simulink subsystem "StudentTemplate_M2_DRAFT3"  (R2025a)
settings: Solver=VariableStepAuto  StartTime=0.0  StopTime=10.0  RelTol=1e-3
libraries: simulink x5, eeGeneralControl x3, slpidlib x3
settings Model: Creator=JesseJabezArendse  LastModifiedBy=MTMTAD006

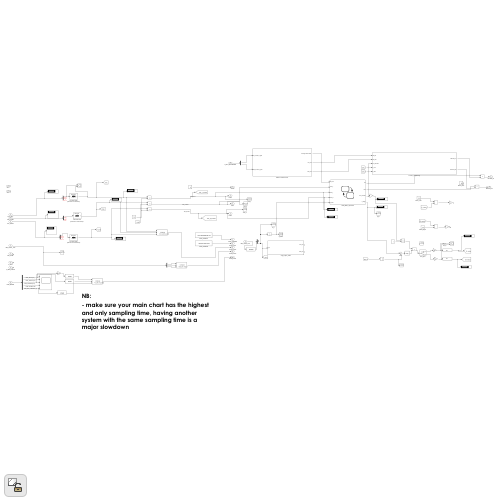
[thumbnail: Simulink's stored preview of the top-level diagram]
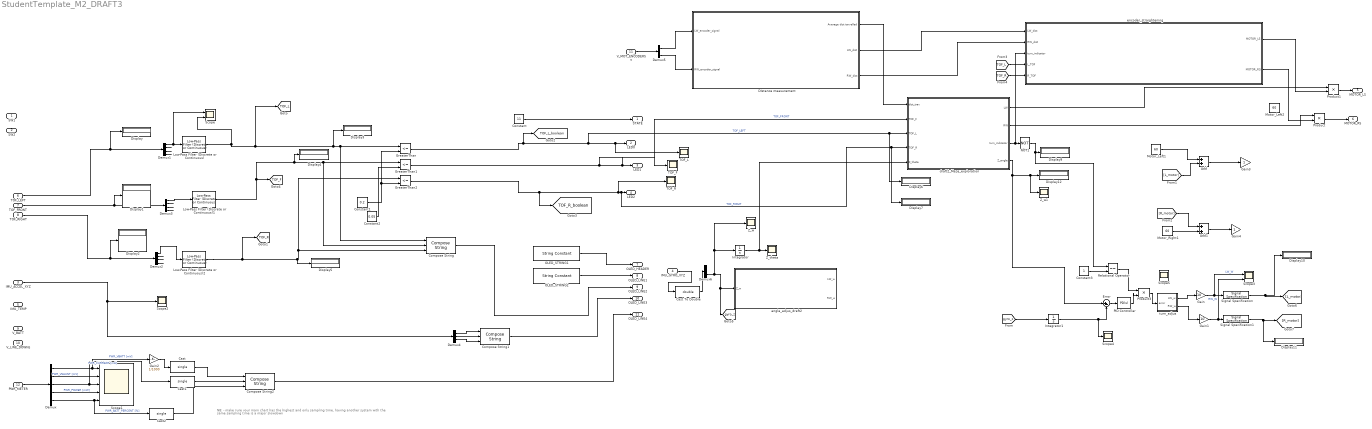
== system StudentTemplate_M2_DRAFT3 ==
  note: NB:
      |
      | - make sure your main chart has the highest and only sampling time, having another system with the same sampling time is a major slowdown
  SW1 : Inport
  SW2 : Inport  Port=2
  IMU_ACCEL_XYZ : Inport  Port=3
  IMU_GYRO_XYZ : Inport  Port=4
  IMU_TEMP : Inport  Port=5
  TOF_LEFT : Inport  Port=6
  TOF_FRONT : Inport  Port=7
  TOF_RIGHT : Inport  Port=8
  V_BATT : Inport  Port=9
  V_LINE_DOWNs : Inport  Port=10
  V_MOT_ENCODERSs : Inport  Port=11
  PWR_METER : Inport  Port=12
  Add : Sum
  Add1 : Sum
  Cast : DataTypeConversion  OutDataTypeStr=single  SaturateOnIntegerOverflow=off  RndMeth=Floor
  Cast To Double : DataTypeConversion  OutDataTypeStr=double  SaturateOnIntegerOverflow=off  RndMeth=Floor
  Cast1 : DataTypeConversion  OutDataTypeStr=single  SaturateOnIntegerOverflow=off  RndMeth=Floor
  Cast2 : DataTypeConversion  OutDataTypeStr=single  SaturateOnIntegerOverflow=off  RndMeth=Floor
  Compose String : ComposeString  Format="\"L%1.2f F%1.2f R%1.2f\""
  Compose String1 : ComposeString  Format="\"X%2.1f  Y%2.1f  Z%2.1f\""
  Compose String2 : ComposeString  Format="\"%1.2fV  %3.0fmA  %2.0f%%\""
  Constant : Constant  Value=11
  Constant1 : Constant  Value=0.2  SampleTime=-1
  Constant2 : Constant  Value=0.05  SampleTime=-1
  Constant3 : Constant
  "DIstance measurement " : Subsystem
  Demux : Demux  Outputs=5
  Demux1 : Demux
  Demux2 : Demux
  Demux3 : Demux
  Demux4 : Demux  Outputs=3
  Demux5 : Demux  Outputs=2
  Demux6 : Demux  Outputs=3
  Display{,1..7,9..12} (12 alike) : Display
  Error : Sum  Inputs=|+-
  Gain : Gain  Gain=10
  Gain1 : Gain  Gain=10
  Gain2 : Gain  Gain=1/1000
  Gain3 : Gain
  Gain4 : Gain
  GreaterThan : RelationalOperator  Operator=<=  OutDataTypeStr=boolean  RndMeth=Simplest  InputSameDT=off
  GreaterThan1 : RelationalOperator  Operator=<=  OutDataTypeStr=boolean  RndMeth=Simplest  InputSameDT=off
  GreaterThan2 : RelationalOperator  Operator=<=  OutDataTypeStr=boolean  RndMeth=Simplest  InputSameDT=off
  Integrator : Integrator
  Integrator1 : Integrator
  Low-Pass Filter (Discrete or Continuous) : eeGeneralControl/Low-Pass Filter (Discrete or Continuous)  K=1  T=0.1  B=inf  A=-inf  init_option=Inherited from block input  x0=0  Ts=-1
  Low-Pass Filter (Discrete or Continuous)1 : eeGeneralControl/Low-Pass Filter (Discrete or Continuous)  K=1  T=0.1  B=inf  A=-inf  init_option=Inherited from block input  x0=0  Ts=-1
  Low-Pass Filter (Discrete or Continuous)2 : eeGeneralControl/Low-Pass Filter (Discrete or Continuous)  K=1  T=0.1  B=inf  A=-inf  init_option=Inherited from block input  x0=0  Ts=-1
  Motor_Left1 : Constant  Value=60
  Motor_Left2 : Constant  Value=60
  Motor_Right1 : Constant  Value=60
  NOT1 : Logic  Operator=NOT  IconShape=distinctive  AllPortsSameDT=off  OutDataTypeStr=boolean
  OLED_STRING1 : StringConstant  String="\"UCT MICROMOUSE '25\""
  OLED_STRING2 : StringConstant  String="\"Simulink Data Demo\""
  PID Controller : slpidlib/PID Controller  Controller=PD  Form=Parallel  TimeDomain=Continuous-time  UseExternalTs=off  SampleTime=-1  IntegratorMethod=Forward Euler  FilterMethod=Forward Euler  ControllerParametersSource=internal  P=50  I=1  UseKiTs=off  D=1  UseExternalDerivativeSource=off  N=100  UseFilter=on  TunerSelectOption=Transfer Function Based (PID Tuner App)  InitialConditionSource=internal  InitialConditionForIntegrator=0  InitialConditionForFilter=0  DifferentiatorICPrevScaledInput=0  ExternalReset=none  TrackingMode=off  Kt=1  LimitOutput=off  SatLimitsSource=internal  UpperSaturationLimit=inf  LowerSaturationLimit=-inf  LinearizeAsGain=on  AntiWindupMode=none  Kb=1  LimitIntegrator=off  UpperIntegratorSaturationLimit=inf  LowerIntegratorSaturationLimit=-inf  POutMin=[]  POutMax=[]  IOutMin=[]  IOutMax=[]  DOutMin=[]  DOutMax=[]  NOutMin=[]  NOutMax=[]  SumOutMin=[]  SumOutMax=[]  SaturationOutMin=[]  SaturationOutMax=[]  PParamMin=[]  PParamMax=[]  IParamMin=[]  IParamMax=[]  DParamMin=[]  DParamMax=[]  NParamMin=[]  NParamMax=[]  KbParamMin=[]  KbParamMax=[]  KtParamMin=[]  KtParamMax=[]  KbOutMin=[]  KbOutMax=[]  KtOutMin=[]  KtOutMax=[]  IntegratorOutMin=[]  IntegratorOutMax=[]  FilterOutMin=[]  FilterOutMax=[]  SumI1OutMin=[]  SumI1OutMax=[]  SumI2OutMin=[]  SumI2OutMax=[]  SumI3OutMin=[]  SumI3OutMax=[]  SumI4OutMin=[]  SumI4OutMax=[]  SumDOutMin=[]  SumDOutMax=[]  DifferentiatorOutMin=[]  DifferentiatorOutMax=[]  FilterDiffOutCoefMin=[]  FilterDiffOutCoefMax=[]  ReciprocalOutMin=[]  ReciprocalOutMax=[]  SumDenOutMin=[]  SumDenOutMax=[]  SumNumOutMin=[]  SumNumOutMax=[]  DivideOutMin=[]  DivideOutMax=[]  UdiffTsProdOutMin=[]  UdiffTsProdOutMax=[]  NTsProdOutMin=[]  NTsProdOutMax=[]  UintegralTsProdOutMin=[]  UintegralTsProdOutMax=[]  UngainTsProdOutMin=[]  UngainTsProdOutMax=[]  ClampingZeroOutDataTypeStr=Inherit: Inherit via back propagation  ClampingZeroOutMin=[]  ClampingZeroOutMax=[]  FilterDenConstantOutDataTypeStr=Inherit: Inherit via back propagation  FilterDenConstantOutMin=[]  FilterDenConstantOutMax=[]  PCopyOutDataTypeStr=Inherit: Inherit via back propagation  PCopyOutMin=[]  PCopyOutMax=[]  NCopyOutDataTypeStr=Inherit: Inherit via back propagation  NCopyOutMin=[]  NCopyOutMax=[]  IntegratorContinuousStateAttributes=''  IntegratorStateMustResolveToSignalObject=off  IntegratorRTWStateStorageClass=Auto  FilterContinuousStateAttributes=''  FilterStateMustResolveToSignalObject=off  FilterRTWStateStorageClass=Auto  ParallelPVariant=InternalParameters  IdealPVariant=Disabled  IVariant=Disabled  DVariant=InternalParameters  IntegratorVariant=Disabled  SatVariant=Disabled  AWVariant=Disabled  PCopyVariant=Disabled  TRVariant=Disabled  FdbkBlocksVariant=Forward  IdealPFdbkVariant=Disabled  SatFdbkVariant=Disabled  DerivativeFilterVariant=ContFilter  NVariant=InternalParameters  NCopyVariant=Disabled  FilterICVariant=InternalICsFilter  IntegratorICVariant=Disabled  ExternalResetVariant=Disabled  TRSumVariant=Passthrough  SumFdbkVariant=Disabled  SumVariant=Sum_PD  TsampFilterVariant=InternalTs  TsampNgainVariant=Passthrough  TsampIntegralVariant=Disabled_SignalSpec  ExternalSaturationOutDataTypeStr=Inherit: Same as second input  DerivativeSourceVariant=ErrorSignal  PreIntVariant=InternalPreInt
  Product : Product
  Product1 : Product
  Product3 : Product
  Relational Operator : RelationalOperator  Operator===  OutDataTypeStr=boolean  RndMeth=Simplest  InputSameDT=off
  Scope : Scope  NumInputPorts=2
      settings: ActiveDisplayYMinimum=0.15223708238283273  ActiveDisplayYMaximum=0.58543478513497516
  Scope1 : Scope  NumInputPorts=5
      settings: ActiveDisplayYMinimum=-437.5  ActiveDisplayYMaximum=3937.5  DataLoggingVariableName=ScopeData2
  Scope2 : Scope
      settings: ActiveDisplayYMinimum=-7.57059273149099  ActiveDisplayYMaximum=14.477362665673041
  Scope3 : Scope  NumInputPorts=2
      settings: ActiveDisplayYMinimum=-440.40684872460486  ActiveDisplayYMaximum=398.93122569343797  DataLoggingVariableName=ScopeData11
  Scope4 : Scope
      settings: ActiveDisplayYMinimum=-2.1976138852237335  ActiveDisplayYMaximum=0.12970641062525379  DataLoggingVariableName=ScopeData14
  Scope5 : Scope
      settings: ActiveDisplayYMinimum=-4.4488284675734473  ActiveDisplayYMaximum=3.9249085751009725  DataLoggingVariableName=ScopeData16
  Signal Specification : SignalSpecification  Dimensions=1
  Signal Specification1 : SignalSpecification  Dimensions=1
  TOF_F : Scope
      settings: ActiveDisplayYMinimum=-0.1769980412947128  ActiveDisplayYMaximum=0.90279895686963285  DataLoggingVariableName=ScopeData4
  TOF_L : Scope
      settings: ActiveDisplayYMinimum=-0.062899688908756052  ActiveDisplayYMaximum=0.13734742485444948  DataLoggingVariableName=ScopeData3
  TOF_R : Scope
      settings: ActiveDisplayYMinimum=0.84085955530656642  ActiveDisplayYMaximum=1.1222796398378163  DataLoggingVariableName=ScopeData5
  Z_theta : Scope
      settings: ActiveDisplayYMinimum=-2.70161604115423  ActiveDisplayYMaximum=4.8892356554264911  DataLoggingVariableName=ScopeData7
  Z_w : Scope
      settings: ActiveDisplayYMinimum=0.15654767663707053  ActiveDisplayYMaximum=0.20860795869615065  DataLoggingVariableName=ScopeData6
  Z_w1 : Scope
      settings: ActiveDisplayYMinimum=0.15654767663707053  ActiveDisplayYMaximum=0.20860795869615065  DataLoggingVariableName=ScopeData25
  angle_adjus_draft2 : Subsystem
  draft2_Maze_exploration : Stateflow chart  TreatAsAtomicUnit=on
      settings: PortSchema="{\"entries\":[{\"content\":{\"sides\":[{\"content\":{\"connectorIds\":[\"In3\",\"In4\",\"In1\",\"In2\",\"In5\"]},\"type\":\"ConnectorPlacement.EquallySpacedRectSide\",\"uuid\":\"48a59af2-7c84-427a-8e2f-b10f2a044ed3\"},{\"content\":{\"connectorIds\":[\"Out1\",\"Out2\",\"Out3\",\"Out4\"],\"side\":\"RIGHT\"},\"type\":\"ConnectorPlacement.EquallySpacedRectSide\",\"uuid\":\"ddb5ed95-9874-42e8-8fee-75458ccb7c53\"},{\"content\":{\"side\":\"TOP\"},\"type\":\"ConnectorPlacement.EquallySpacedRectSide\",\"uuid\":\"d57417fe-864c-49b1-b704-1964fc5ecc42\"}]},\"type\":\"ConnectorPlacement.EquallySpacedConnector\",\"uuid\":\"f24c4a6d-faf6-462a-ab68-e289d44b6927\"}],\"packageUris\":[\"http://schema.mathworks.com/mf0/Connector/R2020b\"],\"version\":\"1.0\"}"
  encoder_straightening : Subsystem
  turn_adjus : Stateflow chart  TreatAsAtomicUnit=on
  STATE : Outport
  LED0 : Outport  Port=2
  LED1 : Outport  Port=3
  LED2 : Outport  Port=4
  MOTOR_LS : Outport  Port=5
  MOTOR_RS : Outport  Port=6
  OLED_HEADER : Outport  Port=7
  OLED_LINE1 : Outport  Port=8
  OLED_LINE2 : Outport  Port=9
  OLED_LINE3 : Outport  Port=10
  OLED_LINE4 : Outport  Port=11
  tag scope: TOF_F=global, TOF_L=global, TOF_L_boolean=global, TOF_R=global, TOF_R_boolean=global, gyro_z=global
  wires:
  TOF_FRONT/1 -> Demux3/1, Display1/1
  OLED_STRING2/1 -> OLED_LINE1/1
  Demux2/1 -> Low-Pass Filter (Discrete or Continuous)2/1
  Demux2/3 -> ?
  Demux2/2 -> ?
  Demux2/4 -> ?
  Compose String1/1 -> OLED_LINE3/1
  Low-Pass Filter (Discrete or Continuous)1/1 -> [TOF_F], Compose String/2, GreaterThan1/1, Display4/1
  GreaterThan1/1 -> LED1/1, TOF_F/1, draft2_Maze_exploration/4(TOF_F)  "TOF_FRONT"
  Demux3/3 -> ?
  TOF_RIGHT/1 -> Demux2/1, Display2/1
  Demux3/4 -> ?
  Demux3/2 -> ?
  Demux1/2 -> ?
  Demux3/1 -> Low-Pass Filter (Discrete or Continuous)1/1
  OLED_STRING1/1 -> OLED_HEADER/1
  Demux1/1 -> Scope/1, Low-Pass Filter (Discrete or Continuous)/1
  Compose String/1 -> OLED_LINE2/1
  Constant1/1 -> GreaterThan2/2, GreaterThan/2
  Demux1/4 -> ?
  GreaterThan2/1 -> TOF_R/1, LED2/1, draft2_Maze_exploration/2(TOF_R), Display7/1, [TOF_R_boolean]  "TOF_RIGHT"
  TOF_LEFT/1 -> Demux1/1, Display/1
  GreaterThan/1 -> LED0/1, TOF_L/1, draft2_Maze_exploration/1(TOF_L), Display6/1, [TOF_L_boolean]  "TOF_LEFT"
  Demux1/3 -> ?
  PWR_METER/1 -> Demux/1
  Demux/1 -> Scope1/1, Gain2/1  "PWR_VBATT [mV]"
  Demux/2 -> Scope1/2  "PWR_VSHUNT [mV]"
  Demux/3 -> Scope1/3, Cast1/1  "PWR_CURRENT [mA]"
  Demux/4 -> Scope1/4  "PWR_POWER [mW]"
  Demux/5 -> Scope1/5, Cast2/1  "PWR_BATT_PERCENT [%]"
  IMU_ACCEL_XYZ/1 -> Demux4/1, Scope2/1
  Demux4/1 -> Compose String1/1
  Demux4/2 -> Compose String1/2
  Demux4/3 -> Compose String1/3
  Compose String2/1 -> OLED_LINE4/1
  Gain2/1 -> Cast/1
  Cast/1 -> Compose String2/1
  Cast1/1 -> Compose String2/2
  Cast2/1 -> Compose String2/3
  Low-Pass Filter (Discrete or Continuous)2/1 -> Compose String/3, GreaterThan2/1, Display5/1, [TOF_R]
  Low-Pass Filter (Discrete or Continuous)/1 -> Scope/2, Compose String/1, GreaterThan/1, Display3/1, [TOF_L]
  Constant/1 -> STATE/1
  V_MOT_ENCODERSs/1 -> Demux5/1
  Demux5/1 -> "DIstance measurement "/1(LW_encoder_signal)
  Demux5/2 -> "DIstance measurement "/2(RW_encoder_signal)
  IMU_GYRO_XYZ/1 -> Cast To Double/1
  Demux6/3 -> angle_adjus_draft2/1(Z_w), [gyro_z], Integrator/1, Z_w/1
  Integrator/1 -> Z_theta/1, draft2_Maze_exploration/5(Z_theta)
  Error/1 -> PID Controller/1
  Signal Specification/1 -> [L_motor], Display10/1
  turn_adjus/1(LW_w) -> Gain/1
  turn_adjus/2(RW_w) -> Gain1/1
  Gain1/1 -> Signal Specification1/1, Scope3/2  "RW_W"
  Integrator1/1 -> Error/2, Scope4/1
  Signal Specification1/1 -> [R_motor], Display11/1
  Gain/1 -> Signal Specification/1, Scope3/1  "LW_W"
  Constant2/1 -> GreaterThan1/2
  draft2_Maze_exploration/1(LW) -> Product1/1
  draft2_Maze_exploration/2(RW) -> Product/1
  Motor_Left1/1 -> Add/1
  Motor_Right1/1 -> Add1/2
  Add/1 -> Gain3/1
  Add1/1 -> Gain4/1
  "DIstance measurement "/1("Average dist tarvelled ") -> draft2_Maze_exploration/3(dist_trav)
  [gyro_z] -> Integrator1/1
  draft2_Maze_exploration/4(Z_angle) -> Error/1, Z_w1/1, Display12/1
  [L_motor] -> Add/2
  [R_motor] -> Add1/1
  draft2_Maze_exploration/3(turn_indicator) -> NOT1/1, encoder_straightening/3(turn_indicator)
  NOT1/1 -> Display9/1, Relational Operator/1
  Constant3/1 -> Relational Operator/2
  PID Controller/1 -> Product3/2
  Product3/1 -> turn_adjus/1(error)
  Relational Operator/1 -> Product3/1
  "DIstance measurement "/2(LW_dist) -> encoder_straightening/1(LW_dist)
  "DIstance measurement "/3(RW_dist) -> encoder_straightening/2(RW_dist)
  [TOF_L] -> encoder_straightening/4(L_TOF)
  [TOF_R] -> encoder_straightening/5(R_TOF)
  Cast To Double/1 -> Demux6/1
  Product1/1 -> MOTOR_LS/1
  Product/1 -> MOTOR_RS/1
  encoder_straightening/1(MOTOR_LS) -> Product1/2
  encoder_straightening/2(MOTOR_RS) -> Product/2

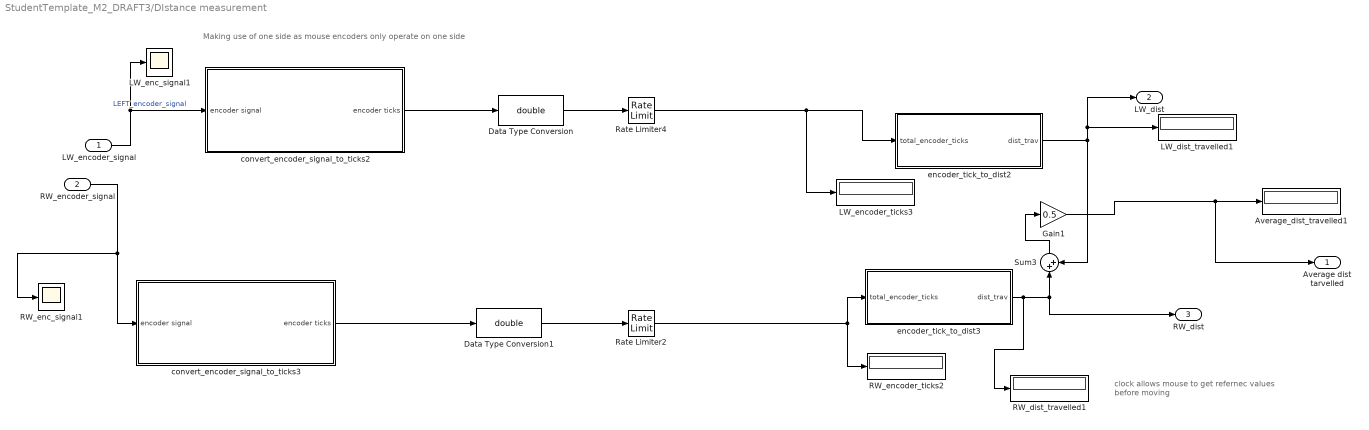
== system StudentTemplate_M2_DRAFT3/DIstance measurement  ==
  note: Making use of one side as mouse encoders only operate on one side
  note: clock allows mouse to get refernec values
      | before moving
  LW_encoder_signal : Inport
  RW_encoder_signal : Inport  Port=2
  Average_dist_travelled1 : Display
  Data Type Conversion : DataTypeConversion  OutDataTypeStr=double  SaturateOnIntegerOverflow=off  RndMeth=Floor
  Data Type Conversion1 : DataTypeConversion  OutDataTypeStr=double  SaturateOnIntegerOverflow=off  RndMeth=Floor
  Gain1 : Gain  Gain=0.5
  LW_dist_travelled1 : Display
  LW_enc_signal1 : Scope
      settings: ActiveDisplayYMinimum=-1.5423087408726712  ActiveDisplayYMaximum=1.7466656009006407  DataLoggingVariableName=ScopeData13
  LW_encoder_ticks3 : Display
  RW_dist_travelled1 : Display
  RW_enc_signal1 : Scope
      settings: ActiveDisplayYMinimum=-1.944570956862778  ActiveDisplayYMaximum=2.0482644886882531  DataLoggingVariableName=ScopeData15
  RW_encoder_ticks2 : Display
  Rate Limiter2 : RateLimiter  RisingSlewLimit=4.85
  Rate Limiter4 : RateLimiter  RisingSlewLimit=4.85
  Sum3 : Sum  Inputs=|++
  convert_encoder_signal_to_ticks2 : Subsystem
  convert_encoder_signal_to_ticks3 : Subsystem
  encoder_tick_to_dist2 : Subsystem
  encoder_tick_to_dist3 : Subsystem
  "Average dist tarvelled " : Outport
  LW_dist : Outport  Port=2
  RW_dist : Outport  Port=3
  wires:
  Data Type Conversion1/1 -> Rate Limiter2/1
  Data Type Conversion/1 -> Rate Limiter4/1
  Rate Limiter2/1 -> RW_encoder_ticks2/1, encoder_tick_to_dist3/1(total_encoder_ticks)
  Rate Limiter4/1 -> encoder_tick_to_dist2/1(total_encoder_ticks), LW_encoder_ticks3/1
  LW_encoder_signal/1 -> convert_encoder_signal_to_ticks2/1(encoder signal), LW_enc_signal1/1  "LEFT_encoder_signal"
  encoder_tick_to_dist3/1(dist_trav) -> RW_dist_travelled1/1, RW_dist/1, Sum3/1
  convert_encoder_signal_to_ticks3/1(encoder ticks) -> Data Type Conversion1/1
  Sum3/1 -> Gain1/1
  convert_encoder_signal_to_ticks2/1(encoder ticks) -> Data Type Conversion/1
  Gain1/1 -> Average_dist_travelled1/1, "Average dist tarvelled "/1
  RW_encoder_signal/1 -> RW_enc_signal1/1, convert_encoder_signal_to_ticks3/1(encoder signal)
  encoder_tick_to_dist2/1(dist_trav) -> Sum3/2, LW_dist_travelled1/1, LW_dist/1

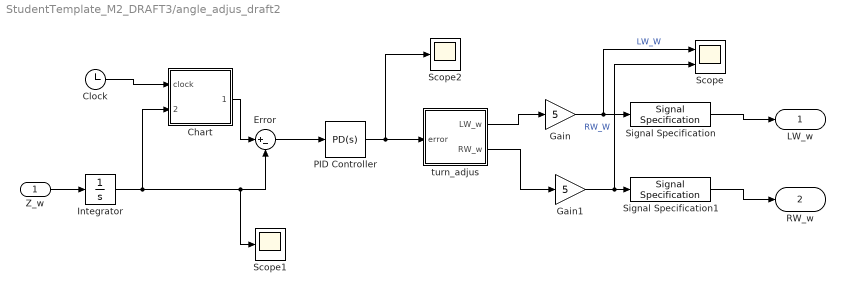
== system StudentTemplate_M2_DRAFT3/angle_adjus_draft2 ==
  Z_w : Inport
  Chart : Stateflow chart  TreatAsAtomicUnit=on
  Clock : Clock
  Error : Sum  Inputs=|+-
  Gain : Gain  Gain=5
  Gain1 : Gain  Gain=5
  Integrator : Integrator
  PID Controller : slpidlib/PID Controller  Controller=PD  Form=Parallel  TimeDomain=Continuous-time  UseExternalTs=off  SampleTime=-1  IntegratorMethod=Forward Euler  FilterMethod=Forward Euler  ControllerParametersSource=internal  P=50  I=1  UseKiTs=off  D=1  UseExternalDerivativeSource=off  N=100  UseFilter=on  TunerSelectOption=Transfer Function Based (PID Tuner App)  InitialConditionSource=internal  InitialConditionForIntegrator=0  InitialConditionForFilter=0  DifferentiatorICPrevScaledInput=0  ExternalReset=none  TrackingMode=off  Kt=1  LimitOutput=off  SatLimitsSource=internal  UpperSaturationLimit=inf  LowerSaturationLimit=-inf  LinearizeAsGain=on  AntiWindupMode=none  Kb=1  LimitIntegrator=off  UpperIntegratorSaturationLimit=inf  LowerIntegratorSaturationLimit=-inf  POutMin=[]  POutMax=[]  IOutMin=[]  IOutMax=[]  DOutMin=[]  DOutMax=[]  NOutMin=[]  NOutMax=[]  SumOutMin=[]  SumOutMax=[]  SaturationOutMin=[]  SaturationOutMax=[]  PParamMin=[]  PParamMax=[]  IParamMin=[]  IParamMax=[]  DParamMin=[]  DParamMax=[]  NParamMin=[]  NParamMax=[]  KbParamMin=[]  KbParamMax=[]  KtParamMin=[]  KtParamMax=[]  KbOutMin=[]  KbOutMax=[]  KtOutMin=[]  KtOutMax=[]  IntegratorOutMin=[]  IntegratorOutMax=[]  FilterOutMin=[]  FilterOutMax=[]  SumI1OutMin=[]  SumI1OutMax=[]  SumI2OutMin=[]  SumI2OutMax=[]  SumI3OutMin=[]  SumI3OutMax=[]  SumI4OutMin=[]  SumI4OutMax=[]  SumDOutMin=[]  SumDOutMax=[]  DifferentiatorOutMin=[]  DifferentiatorOutMax=[]  FilterDiffOutCoefMin=[]  FilterDiffOutCoefMax=[]  ReciprocalOutMin=[]  ReciprocalOutMax=[]  SumDenOutMin=[]  SumDenOutMax=[]  SumNumOutMin=[]  SumNumOutMax=[]  DivideOutMin=[]  DivideOutMax=[]  UdiffTsProdOutMin=[]  UdiffTsProdOutMax=[]  NTsProdOutMin=[]  NTsProdOutMax=[]  UintegralTsProdOutMin=[]  UintegralTsProdOutMax=[]  UngainTsProdOutMin=[]  UngainTsProdOutMax=[]  ClampingZeroOutDataTypeStr=Inherit: Inherit via back propagation  ClampingZeroOutMin=[]  ClampingZeroOutMax=[]  FilterDenConstantOutDataTypeStr=Inherit: Inherit via back propagation  FilterDenConstantOutMin=[]  FilterDenConstantOutMax=[]  PCopyOutDataTypeStr=Inherit: Inherit via back propagation  PCopyOutMin=[]  PCopyOutMax=[]  NCopyOutDataTypeStr=Inherit: Inherit via back propagation  NCopyOutMin=[]  NCopyOutMax=[]  IntegratorContinuousStateAttributes=''  IntegratorStateMustResolveToSignalObject=off  IntegratorRTWStateStorageClass=Auto  FilterContinuousStateAttributes=''  FilterStateMustResolveToSignalObject=off  FilterRTWStateStorageClass=Auto  ParallelPVariant=InternalParameters  IdealPVariant=Disabled  IVariant=Disabled  DVariant=InternalParameters  IntegratorVariant=Disabled  SatVariant=Disabled  AWVariant=Disabled  PCopyVariant=Disabled  TRVariant=Disabled  FdbkBlocksVariant=Forward  IdealPFdbkVariant=Disabled  SatFdbkVariant=Disabled  DerivativeFilterVariant=ContFilter  NVariant=InternalParameters  NCopyVariant=Disabled  FilterICVariant=InternalICsFilter  IntegratorICVariant=Disabled  ExternalResetVariant=Disabled  TRSumVariant=Passthrough  SumFdbkVariant=Disabled  SumVariant=Sum_PD  TsampFilterVariant=InternalTs  TsampNgainVariant=Passthrough  TsampIntegralVariant=Disabled_SignalSpec  ExternalSaturationOutDataTypeStr=Inherit: Same as second input  DerivativeSourceVariant=ErrorSignal  PreIntVariant=InternalPreInt
  Scope : Scope  NumInputPorts=2
      settings: ActiveDisplayYMinimum=-440.40684872460486  ActiveDisplayYMaximum=398.93122569343797  DataLoggingVariableName=ScopeData8
  Scope1 : Scope
      settings: ActiveDisplayYMinimum=-2.1976138852237335  ActiveDisplayYMaximum=0.12970641062525379  DataLoggingVariableName=ScopeData12
  Scope2 : Scope
      settings: ActiveDisplayYMinimum=-4.4488284675734473  ActiveDisplayYMaximum=3.9249085751009725  DataLoggingVariableName=ScopeData10
  Signal Specification : SignalSpecification  Dimensions=1
  Signal Specification1 : SignalSpecification  Dimensions=1
  turn_adjus : Stateflow chart  TreatAsAtomicUnit=on
  LW_w : Outport
  RW_w : Outport  Port=2
  wires:
  Clock/1 -> Chart/1(clock)
  Gain1/1 -> Signal Specification1/1, Scope/2  "RW_W"
  Gain/1 -> Signal Specification/1, Scope/1  "LW_W"
  Chart/1(offset) -> Error/1
  Z_w/1 -> Integrator/1
  Signal Specification1/1 -> RW_w/1
  Signal Specification/1 -> LW_w/1
  turn_adjus/2(RW_w) -> Gain1/1
  turn_adjus/1(LW_w) -> Gain/1
  PID Controller/1 -> turn_adjus/1(error), Scope2/1
  Error/1 -> PID Controller/1
  Integrator/1 -> Error/2, Scope1/1, Chart/2(Z_theta)

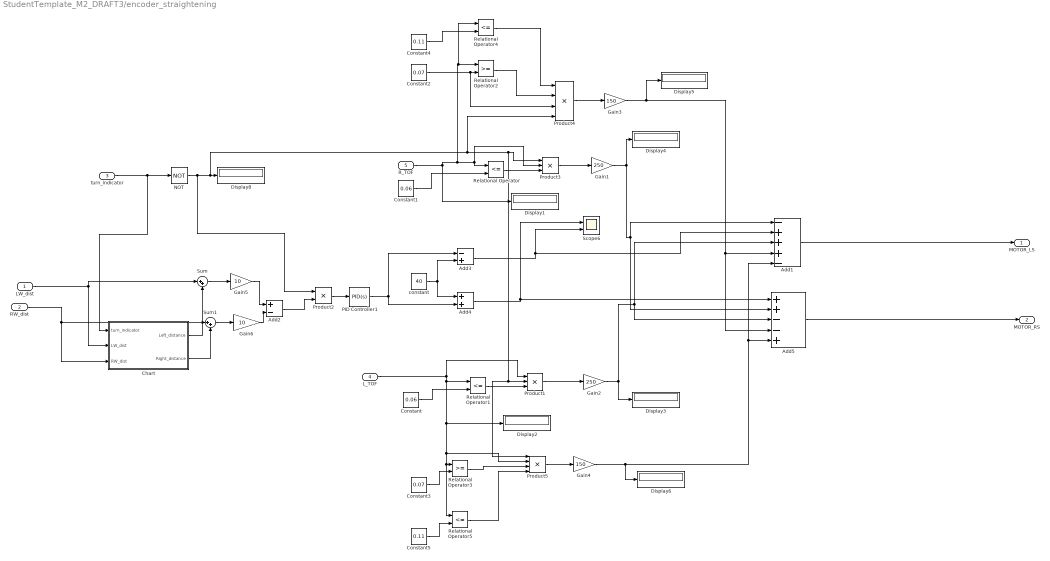
== system StudentTemplate_M2_DRAFT3/encoder_straightening ==
  LW_dist : Inport
  RW_dist : Inport  Port=2
  turn_indicator : Inport  Port=3
  L_TOF : Inport  Port=4
  R_TOF : Inport  Port=5
  Add1 : Sum  Inputs=-+++-
  Add2 : Sum  Inputs=+-
  Add3 : Sum  Inputs=-+
  Add4 : Sum
  Add5 : Sum  Inputs=++--+
  Chart : Stateflow chart  TreatAsAtomicUnit=on
      settings: PortSchema="{\"entries\":[{\"content\":{\"sides\":[{\"content\":{\"connectorIds\":[\"In1\",\"In3\",\"In2\"]},\"type\":\"ConnectorPlacement.EquallySpacedRectSide\",\"uuid\":\"fc51768e-ed5b-46a0-b3fc-5b0af41a010d\"},{\"content\":{\"connectorIds\":[\"Out1\",\"Out2\"],\"side\":\"RIGHT\"},\"type\":\"ConnectorPlacement.EquallySpacedRectSide\",\"uuid\":\"30fd33ca-4b93-4317-9d26-1d1e6ba5d493\"},{\"content\":{\"side\":\"TOP\"},\"type\":\"ConnectorPlacement.EquallySpacedRectSide\",\"uuid\":\"029c60dd-f0f8-450d-b3c4-7fca568cb539\"}]},\"type\":\"ConnectorPlacement.EquallySpacedConnector\",\"uuid\":\"245ec1db-d65a-48a6-a1e3-28a0f03f23bc\"}],\"packageUris\":[\"http://schema.mathworks.com/mf0/Connector/R2020b\"],\"version\":\"1.0\"}"
  Constant : Constant  Value=0.06
  Constant1 : Constant  Value=0.06
  Constant2 : Constant  Value=0.07
  Constant3 : Constant  Value=0.07
  Constant4 : Constant  Value=0.11
  Constant5 : Constant  Value=0.11
  Display{1..6,8} (7 alike) : Display
  Gain1 : Gain  Gain=250
  Gain2 : Gain  Gain=250
  Gain3 : Gain  Gain=150
  Gain4 : Gain  Gain=150
  Gain5 : Gain  Gain=10
  Gain6 : Gain  Gain=10
  NOT : Logic  Operator=NOT  IconShape=distinctive  AllPortsSameDT=off  OutDataTypeStr=boolean
  PID Controller1 : slpidlib/PID Controller  Controller=PID  Form=Parallel  TimeDomain=Continuous-time  UseExternalTs=off  SampleTime=-1  IntegratorMethod=Forward Euler  FilterMethod=Forward Euler  ControllerParametersSource=internal  P=75  I=1  UseKiTs=off  D=0  UseExternalDerivativeSource=off  N=100  UseFilter=on  TunerSelectOption=Transfer Function Based (PID Tuner App)  InitialConditionSource=internal  InitialConditionForIntegrator=0  InitialConditionForFilter=0  DifferentiatorICPrevScaledInput=0  ExternalReset=none  TrackingMode=off  Kt=1  LimitOutput=off  SatLimitsSource=internal  UpperSaturationLimit=inf  LowerSaturationLimit=-inf  LinearizeAsGain=on  AntiWindupMode=none  Kb=1  LimitIntegrator=off  UpperIntegratorSaturationLimit=inf  LowerIntegratorSaturationLimit=-inf  POutMin=[]  POutMax=[]  IOutMin=[]  IOutMax=[]  DOutMin=[]  DOutMax=[]  NOutMin=[]  NOutMax=[]  SumOutMin=[]  SumOutMax=[]  SaturationOutMin=[]  SaturationOutMax=[]  PParamMin=[]  PParamMax=[]  IParamMin=[]  IParamMax=[]  DParamMin=[]  DParamMax=[]  NParamMin=[]  NParamMax=[]  KbParamMin=[]  KbParamMax=[]  KtParamMin=[]  KtParamMax=[]  KbOutMin=[]  KbOutMax=[]  KtOutMin=[]  KtOutMax=[]  IntegratorOutMin=[]  IntegratorOutMax=[]  FilterOutMin=[]  FilterOutMax=[]  SumI1OutMin=[]  SumI1OutMax=[]  SumI2OutMin=[]  SumI2OutMax=[]  SumI3OutMin=[]  SumI3OutMax=[]  SumI4OutMin=[]  SumI4OutMax=[]  SumDOutMin=[]  SumDOutMax=[]  DifferentiatorOutMin=[]  DifferentiatorOutMax=[]  FilterDiffOutCoefMin=[]  FilterDiffOutCoefMax=[]  ReciprocalOutMin=[]  ReciprocalOutMax=[]  SumDenOutMin=[]  SumDenOutMax=[]  SumNumOutMin=[]  SumNumOutMax=[]  DivideOutMin=[]  DivideOutMax=[]  UdiffTsProdOutMin=[]  UdiffTsProdOutMax=[]  NTsProdOutMin=[]  NTsProdOutMax=[]  UintegralTsProdOutMin=[]  UintegralTsProdOutMax=[]  UngainTsProdOutMin=[]  UngainTsProdOutMax=[]  ClampingZeroOutDataTypeStr=Inherit: Inherit via back propagation  ClampingZeroOutMin=[]  ClampingZeroOutMax=[]  FilterDenConstantOutDataTypeStr=Inherit: Inherit via back propagation  FilterDenConstantOutMin=[]  FilterDenConstantOutMax=[]  PCopyOutDataTypeStr=Inherit: Inherit via back propagation  PCopyOutMin=[]  PCopyOutMax=[]  NCopyOutDataTypeStr=Inherit: Inherit via back propagation  NCopyOutMin=[]  NCopyOutMax=[]  IntegratorContinuousStateAttributes=''  IntegratorStateMustResolveToSignalObject=off  IntegratorRTWStateStorageClass=Auto  FilterContinuousStateAttributes=''  FilterStateMustResolveToSignalObject=off  FilterRTWStateStorageClass=Auto  ParallelPVariant=InternalParameters  IdealPVariant=Disabled  IVariant=InternalParameters  DVariant=InternalParameters  IntegratorVariant=Continuous  SatVariant=Disabled  AWVariant=Passthrough  PCopyVariant=Disabled  TRVariant=Disabled  FdbkBlocksVariant=Forward  IdealPFdbkVariant=Disabled  SatFdbkVariant=Disabled  DerivativeFilterVariant=ContFilter  NVariant=InternalParameters  NCopyVariant=Disabled  FilterICVariant=InternalICsFilter  IntegratorICVariant=InternalICs  ExternalResetVariant=Disabled  TRSumVariant=Passthrough  SumFdbkVariant=Disabled  SumVariant=Sum_PID  TsampFilterVariant=InternalTs  TsampNgainVariant=Passthrough  TsampIntegralVariant=Disabled_SignalSpec  ExternalSaturationOutDataTypeStr=Inherit: Same as second input  DerivativeSourceVariant=ErrorSignal  PreIntVariant=InternalPreInt
  Product1 : Product  Inputs=3
  Product2 : Product
  Product3 : Product  Inputs=3
  Product4 : Product  Inputs=4
  Product5 : Product  Inputs=4
  Relational Operator{,1,4..5} (4 alike) : RelationalOperator  Operator=<=  OutDataTypeStr=boolean  RndMeth=Simplest  InputSameDT=off
  Relational Operator2 : RelationalOperator  OutDataTypeStr=boolean  RndMeth=Simplest  InputSameDT=off
  Relational Operator3 : RelationalOperator  OutDataTypeStr=boolean  RndMeth=Simplest  InputSameDT=off
  Scope6 : Scope  NumInputPorts=2
      settings: ActiveDisplayYMinimum=-0.00015132169145948109  ActiveDisplayYMaximum=8.2179160600609662E-5  DataLoggingVariableName=ScopeData24
  Sum : Sum  Inputs=|++
  Sum1 : Sum  Inputs=|++
  constant : Constant  Value=40
  MOTOR_LS : Outport
  MOTOR_RS : Outport  Port=2
  wires:
  Relational Operator5/1 -> Product5/4
  Constant5/1 -> Relational Operator5/2
  Relational Operator4/1 -> Product4/1
  Constant4/1 -> Relational Operator4/2
  Gain4/1 -> Add5/5, Add1/5, Display6/1
  Product5/1 -> Gain4/1
  Relational Operator3/1 -> Product5/3
  Constant3/1 -> Relational Operator3/2
  Gain3/1 -> Add1/4, Add5/4, Display5/1
  Product4/1 -> Gain3/1
  Relational Operator2/1 -> Product4/2
  Constant2/1 -> Relational Operator2/2, Product4/3
  Gain1/1 -> Display4/1, Add1/1, Add5/2
  Gain2/1 -> Display3/1, Add5/3, Add1/3
  Add5/1 -> MOTOR_RS/1
  Product1/1 -> Gain2/1
  Add1/1 -> MOTOR_LS/1
  Product3/1 -> Gain1/1
  Constant1/1 -> Relational Operator/2
  Relational Operator/1 -> Product3/3
  Relational Operator1/1 -> Product1/3
  Constant/1 -> Relational Operator1/2
  L_TOF/1 -> Product1/1, Display2/1, Relational Operator3/1, Relational Operator5/1, Product5/2, Relational Operator1/1
  R_TOF/1 -> Display1/1, Relational Operator/1, Product3/2, Relational Operator2/1, Relational Operator4/1
  Chart/2(Right_distance) -> Sum1/2
  Sum1/1 -> Gain6/1
  Chart/1(Left_distance) -> Sum/2
  Sum/1 -> Gain5/1
  NOT/1 -> Display8/1, Product3/1, Product5/1, Product1/2, Product4/4, Product2/1
  RW_dist/1 -> Chart/2(RW_dist), Sum1/1
  LW_dist/1 -> Sum/1, Chart/3(LW_dist)
  turn_indicator/1 -> NOT/1, Chart/1(turn_indicator)
  Gain6/1 -> Add2/2
  PID Controller1/1 -> Add4/2, Add3/1
  Add2/1 -> Product2/2
  constant/1 -> Add4/1, Add3/2
  Product2/1 -> PID Controller1/1
  Add3/1 -> Add1/2, Scope6/2
  Gain5/1 -> Add2/1
  Add4/1 -> Add5/1, Scope6/1

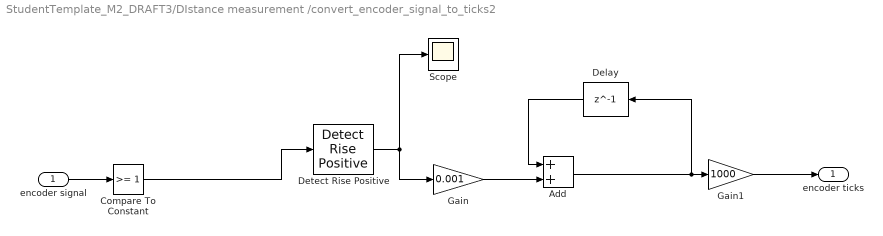
== system StudentTemplate_M2_DRAFT3/DIstance measurement /convert_encoder_signal_to_ticks2 ==
  encoder signal : Inport
  Add : Sum
  Compare To Constant : simulink/Logic and Bit Operations/Compare To Constant  relop=>=  const=1  OutDataTypeStr=boolean
  Delay : Delay  DelayLength=1  InitialCondition=0
  Detect Rise Positive : simulink/Logic and Bit Operations/Detect Rise Positive  vinit=0  OutDataTypeStr=uint8
  Gain : Gain  Gain=0.001
  Gain1 : Gain  Gain=1000
  Scope : Scope
      settings: ActiveDisplayYMinimum=-0.30381603839463822  ActiveDisplayYMaximum=1.4550594899256748  DataLoggingVariableName=ScopeData9
  encoder ticks : Outport
  wires:
  Gain1/1 -> encoder ticks/1
  Gain/1 -> Add/2
  Add/1 -> Gain1/1, Delay/1
  Compare To Constant/1 -> Detect Rise Positive/1
  Detect Rise Positive/1 -> Gain/1, Scope/1
  encoder signal/1 -> Compare To Constant/1
  Delay/1 -> Add/1

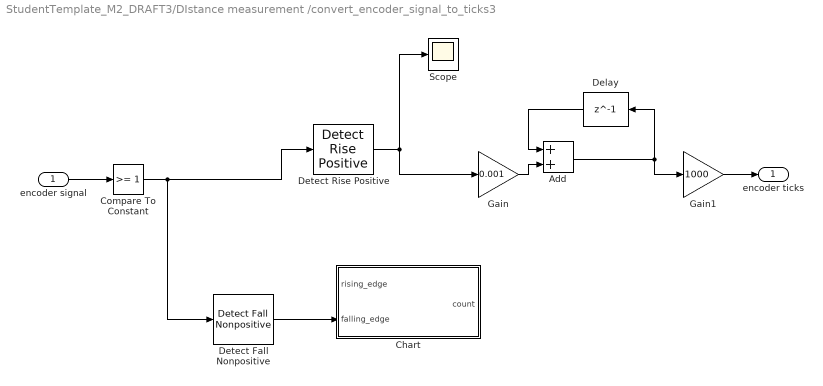
== system StudentTemplate_M2_DRAFT3/DIstance measurement /convert_encoder_signal_to_ticks3 ==
  encoder signal : Inport
  Add : Sum
  Chart : Stateflow chart  TreatAsAtomicUnit=on
  Compare To Constant : simulink/Logic and Bit Operations/Compare To Constant  relop=>=  const=1  OutDataTypeStr=boolean
  Delay : Delay  DelayLength=1  InitialCondition=0
  Detect Fall Nonpositive : simulink/Logic and Bit Operations/Detect Fall Nonpositive  vinit=0  OutDataTypeStr=boolean
  Detect Rise Positive : simulink/Logic and Bit Operations/Detect Rise Positive  vinit=0  OutDataTypeStr=uint8
  Gain : Gain  Gain=0.001
  Gain1 : Gain  Gain=1000
  Scope : Scope
      settings: ActiveDisplayYMinimum=-0.30381603839463822  ActiveDisplayYMaximum=1.4550594899256748  DataLoggingVariableName=ScopeData9
  encoder ticks : Outport
  wires:
  Gain1/1 -> encoder ticks/1
  Gain/1 -> Add/2
  Add/1 -> Delay/1, Gain1/1
  Compare To Constant/1 -> Detect Fall Nonpositive/1, Detect Rise Positive/1
  Detect Rise Positive/1 -> Gain/1, Scope/1
  encoder signal/1 -> Compare To Constant/1
  Delay/1 -> Add/1
  Detect Fall Nonpositive/1 -> Chart/2(falling_edge)

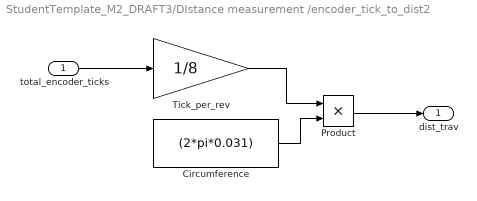
== system StudentTemplate_M2_DRAFT3/DIstance measurement /encoder_tick_to_dist2 ==
  total_encoder_ticks : Inport
  Circumference : Constant  Value=(2*pi*0.031)
  Product : Product
  Tick_per_rev : Gain  Gain=1/8
  dist_trav : Outport
  wires:
  Product/1 -> dist_trav/1
  Tick_per_rev/1 -> Product/1
  Circumference/1 -> Product/2
  total_encoder_ticks/1 -> Tick_per_rev/1

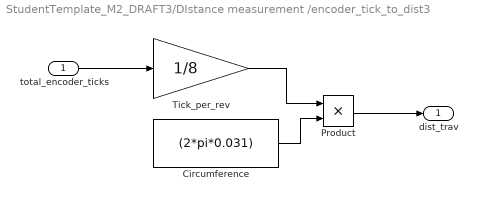
== system StudentTemplate_M2_DRAFT3/DIstance measurement /encoder_tick_to_dist3 ==
  total_encoder_ticks : Inport
  Circumference : Constant  Value=(2*pi*0.031)
  Product : Product
  Tick_per_rev : Gain  Gain=1/8
  dist_trav : Outport
  wires:
  Product/1 -> dist_trav/1
  Tick_per_rev/1 -> Product/1
  Circumference/1 -> Product/2
  total_encoder_ticks/1 -> Tick_per_rev/1

== stateflow chart StudentTemplate_M2_DRAFT3/angle_adjus_draft2/turn_adjus ==
  state deafult
    during:
    LW_w = 0;
    RW_w = 0;
  state turnLeft
    during:
    LW_w=-error;
    RW_w = error;
  state turnRight
    during:
    RW_w = error;
    LW_w = -error;
  (default) -> deafult
  deafult -> turnLeft [order 2] : [error>0 ]
  deafult -> turnRight [order 1] : [error<0 ]
  data: error input; LW_w output; RW_w output

== stateflow chart StudentTemplate_M2_DRAFT3/angle_adjus_draft2/Chart ==
  state Start
    during:
    offset= 0;
  state Set_Offset
    during:
    offset = Z_theta;
  (default) -> Start
  Start -> Set_Offset : [clock <0.1]
  Set_Offset -> Set_Offset : [clock > 0.1]
  data: clock input; offset output; Z_theta input

== stateflow chart StudentTemplate_M2_DRAFT3/turn_adjus ==
  state deafult
    during:
    LW_w = 0;
    RW_w = 0;
  state turnLeft
    during:
    LW_w=-error;
    RW_w = error;
  state turnRight
    during:
    RW_w = error;
    LW_w = -error;
  (default) -> deafult
  deafult -> turnLeft [order 2] : [error>0 ]
  deafult -> turnRight [order 1] : [error<0 ]
  data: error input; LW_w output; RW_w output

== stateflow chart StudentTemplate_M2_DRAFT3/DIstance measurement /convert_encoder_signal_to_ticks3/Chart ==
  state default
    during:
    count =0;
  state encoder_pulse_start
    during:
  state encoder_pulse_end
    during:
    count = 1;
  (default) -> default
  default -> encoder_pulse_start : [rising_edge == 1]
  encoder_pulse_start -> encoder_pulse_end : [falling_edge == 1]
  data: rising_edge input; count output; falling_edge input

== stateflow chart StudentTemplate_M2_DRAFT3/draft2_Maze_exploration ==
  settings: updateMethod=CONTINUOUS  sampleTime=0.005
  state Left_turn1
    entry:
    theta = Z_theta;
    Z_angle = Z_angle +pi/2;
    turn_dist = dist_trav;
    turn_dist = turn_dist +(0.055 *pi/2);
    during:
    LW = -1;
    RW = 1;
    exit:
    turn_indicator = 1
  state Go_straight
    during:
    LW = 1;
    RW = 1;
  state left_turn_setup
    entry:
    start_dist = dist_trav;
    end_dist = start_dist + 0.14;
  state Go_straight1
    entry:
    turn_indicator = 0;
    during:
    LW = 1;
    RW = 1;
  state set_Z_angle
    entry:
    Z_angle = 0;
    LW = 0;
    RW = 0;
  state Start
    entry:
    LW = 0;
    RW =0;
    turn_indicator = 0;
  state Left_turn
    entry:
    theta = Z_theta;
    Z_angle = Z_angle + pi/2;
    turn_dist = dist_trav;
    turn_dist = turn_dist +(0.055 *pi/2);
    during:
    LW = -1;
    RW = 1;
    exit:
    turn_indicator = 1;
  state Full_rotation
    entry:
    theta = Z_theta;
    Z_angle = Z_angle - pi;
    during:
    LW = 1;
    RW =-1;
    exit:
    turn_indicator = 1;
  state Left_turn2
    entry:
    theta = Z_theta;
    Z_angle = Z_angle +pi/2;
    turn_dist = dist_trav;
    turn_dist = turn_dist +(0.055 *pi/2);
    during:
    LW = -1;
    RW = 1;
    exit:
    turn_indicator = 1;
  state left_turn_setup1
    entry:
    start_dist = dist_trav;
    end_dist = start_dist + 0.14;
  state right_turn
    entry:
    theta =Z_theta;
    Z_angle = Z_angle - pi/2;
    turn_dist = dist_trav;
    turn_dist = turn_dist +(0.055 *pi/2);
    during:
    LW = 1;
    RW =-1;
    exit:
    turn_indicator = 1;
  left_turn_setup -> Left_turn1 [order 2] : [dist_trav >= end_dist  || TOF_F == 1 && TOF_L == 0 ]
  Go_straight -> left_turn_setup [order 2] : [TOF_F ==0 && TOF_L ==0]
  Start -> Go_straight [order 4] : [TOF_L == 1 && TOF_F == 0 || TOF_R == 1 && TOF_F ==0]
  Go_straight -> (junction 107) [order 1] : [TOF_F ==1  ]
  Left_turn1 -> Go_straight1 : [dist_trav >= turn_dist && Z_theta >= Z_angle  ]
  left_turn_setup -> (junction 103) [order 1] : [TOF_L ==1 ]
  (default) -> set_Z_angle
  (junction 103) -> (junction 107)
  Go_straight1 -> (junction 103) [order 1] : [TOF_F ==1  ]
  left_turn_setup1 -> (junction 103) [order 1] : [TOF_L ==1 ]
  (junction 107) -> Start
  Full_rotation -> (junction 103) : [Z_theta <= Z_angle && TOF_F == 0 ]
  Go_straight1 -> left_turn_setup1 [order 2] : [TOF_F ==0 && TOF_L ==0]
  set_Z_angle -> Start
  Start -> Full_rotation [order 1] : [TOF_L == 1 && TOF_R == 1 && TOF_F ==1]
  Start -> Left_turn [order 2] : [TOF_L ==0 && TOF_F ==1]
  Left_turn2 -> Start : [Z_theta >= Z_angle && dist_trav >= turn_dist]
  Left_turn -> Start : [Z_theta >= Z_angle && dist_trav >= turn_dist]
  right_turn -> Start : [Z_theta <= Z_angle && dist_trav >= turn_dist]
  Start -> right_turn [order 3] : [TOF_R ==0 && TOF_F ==1]
  left_turn_setup1 -> Left_turn2 [order 2] : [dist_trav >= end_dist || TOF_F == 1 && TOF_L == 0  ]
  data: TOF_L input; TOF_R input; LW output; RW output; dist_trav input; start_dist local; TOF_F input; end_dist local; Z_theta input; turn_indicator output; theta local; Z_angle output; turn_dist local

== stateflow chart StudentTemplate_M2_DRAFT3/encoder_straightening/Chart ==
  state after_turn
    entry:
    during:
    if (LW_dist > RW_dist)
    Right_distance = difference;
    elseif (RW_dist > LW_dist)
    Left_distance =  difference;
    end
  state distance_corrcetion
    exit:
    difference = RW_dist - LW_dist;
    difference = abs(difference)
  (default) -> distance_corrcetion
  after_turn -> distance_corrcetion : [turn_indicator == 1]
  distance_corrcetion -> after_turn : [turn_indicator == 0]
  data: turn_indicator input; RW_dist input; Left_distance output; LW_dist input; Right_distance output; difference local
